simulink model "maglev"  (R2024a)
settings: Solver=VariableStepAuto  StartTime=0.0  StopTime=10.0  RelTol=1e-3
values from neighbouring files (symbols this model uses):
  A = 0    [maglev_parameters.m]
  Cd = 0    [maglev_parameters.m]
  g = 9.81    [maglev_parameters.m]
  m = 0.06157    [maglev_parameters.m]
  R1 = 150    [maglev_parameters.m]
  R2 = 150    [maglev_parameters.m]
  rho = 0    [maglev_parameters.m]
  v0 = 0    [maglev_parameters.m]
  z0 = 0.01    [maglev_parameters.m]
settings Model: Creator=Bocchio  LastModifiedBy=Bocchio

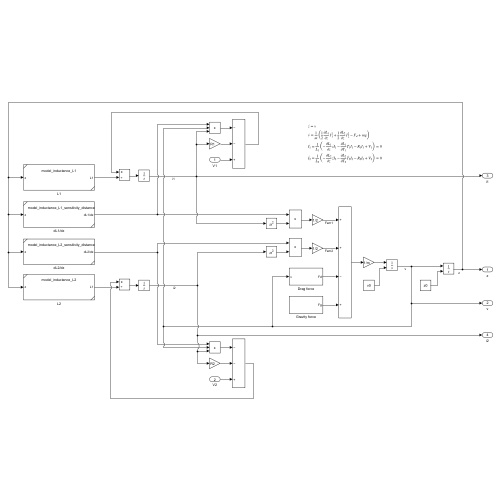
[thumbnail: Simulink's stored preview of the top-level diagram]
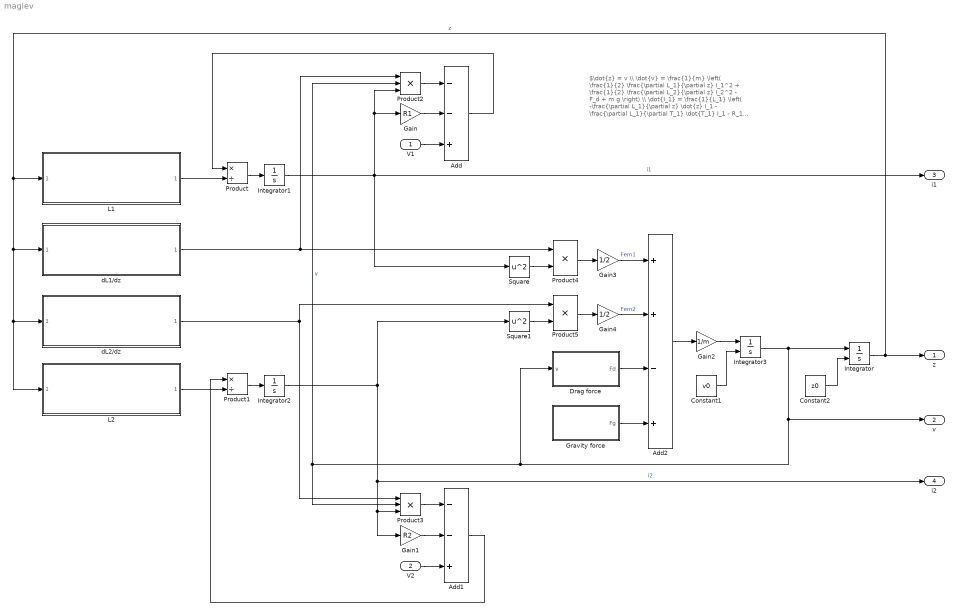
== system maglev ==
  note: $\dot{z} = v \\ \dot{v} = \frac{1}{m} \left( \frac{1}{2} \frac{\partial L_1}{\partial z} I_1^2 + \frac{1}{2} \frac{\partial L_2}{\partial z} I_2^2 - F_d + m g \right) \\ \dot{I_1} = \frac{1}{L_1} \left( -\frac{\partial L_1}{\partial z} \dot{z} I_1 - \frac{\partial L_1}{\partial T_1} \dot{T_1} I_1 - R_1 I_1 + V_1 \right) = 0 \\ \dot{I_2} = \frac{1}{L_2} \left( -\frac{\partial L_2}{\partial z} \dot{z} I_2 - \frac{\partial L_2}{\partial T_2} \dot{T_2} I_2 - R_2 I_2 + V_2 \right) = 0$
  V1 : Inport
  V2 : Inport  Port=2
  Add : Sum  Inputs=--+
  Add1 : Sum  Inputs=--+
  Add2 : Sum  Inputs=++-+
  Constant1 : Constant  Value=v0
  Constant2 : Constant  Value=z0
  Drag force : Subsystem
  Gain : Gain  Gain=R1
  Gain1 : Gain  Gain=R2
  Gain2 : Gain  Gain=1/m
  Gain3 : Gain  Gain=1/2
  Gain4 : Gain  Gain=1/2
  Gravity force : Subsystem
  Integrator : Integrator  InitialConditionSource=external
  Integrator1 : Integrator
  Integrator2 : Integrator
  Integrator3 : Integrator  InitialConditionSource=external
  L1 : Subsystem  ReferencedSubsystem=model_inductance_L1
  L2 : Subsystem  ReferencedSubsystem=model_inductance_L2
  Product : Product  Inputs=*/
  Product1 : Product  Inputs=*/
  Product2 : Product  Inputs=3
  Product3 : Product  Inputs=3
  Product4 : Product
  Product5 : Product
  Square : Math  Operator=square
  Square1 : Math  Operator=square
  dL1/dz : Subsystem  ReferencedSubsystem=model_inductance_L1_sensitivity_distance
  dL2/dz : Subsystem  ReferencedSubsystem=model_inductance_L2_sensitivity_distance
  z : Outport
  v : Outport  Port=2
  i1 : Outport  Port=3
  i2 : Outport  Port=4
  wires:
  Integrator/1 -> z/1, dL2/dz/1, L2/1, dL1/dz/1, L1/1  "z"
  dL1/dz/1 -> Product4/1, Product2/1
  Add1/1 -> Product1/1
  Gain3/1 -> Add2/1  "Fem1"
  Product3/1 -> Add1/1
  dL2/dz/1 -> Product5/1, Product3/1
  Product/1 -> Integrator1/1
  Product2/1 -> Add/1
  Product1/1 -> Integrator2/1
  Gain4/1 -> Add2/2  "Fem2"
  Square/1 -> Product4/2
  Square1/1 -> Product5/2
  Integrator1/1 -> Square/1, i1/1, Product2/3, Gain/1  "i1"
  Add2/1 -> Gain2/1
  Product4/1 -> Gain3/1
  L1/1 -> Product/2
  Product5/1 -> Gain4/1
  Integrator3/1 -> Product2/2, Product3/2, Drag force/1(v), v/1, Integrator/1  "v"
  Integrator2/1 -> i2/1, Gain1/1, Product3/3, Square1/1  "i2"
  V1/1 -> Add/3
  Add/1 -> Product/1
  Gain/1 -> Add/2
  Drag force/1(Fd) -> Add2/3
  Gain1/1 -> Add1/2
  V2/1 -> Add1/3
  Gain2/1 -> Integrator3/1
  L2/1 -> Product1/2
  Constant1/1 -> Integrator3/2
  Constant2/1 -> Integrator/2
  Gravity force/1(Fg) -> Add2/4

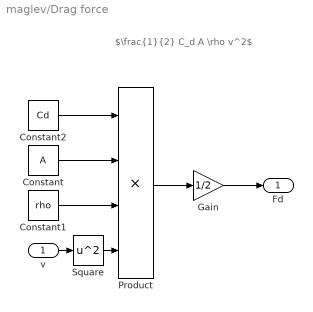
== system maglev/Drag force ==
  note: $\frac{1}{2} C_d A \rho v^2$
  v : Inport
  Constant : Constant  Value=A
  Constant1 : Constant  Value=rho
  Constant2 : Constant  Value=Cd
  Gain : Gain  Gain=1/2
  Product : Product  Inputs=4
  Square : Math  Operator=square
  Fd : Outport
  wires:
  Constant1/1 -> Product/3
  Constant/1 -> Product/2
  Constant2/1 -> Product/1
  Gain/1 -> Fd/1
  Product/1 -> Gain/1
  v/1 -> Square/1
  Square/1 -> Product/4

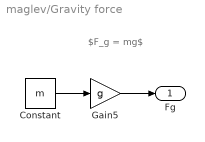
== system maglev/Gravity force ==
  note: $F_g = mg$
  Constant : Constant  Value=m
  Gain5 : Gain  Gain=g
  Fg : Outport
  wires:
  Gain5/1 -> Fg/1
  Constant/1 -> Gain5/1
